simulink model "InverterOnly"  (R2016b)
settings: Solver=ode45  StartTime=0*24*3600  StopTime=3600  MaxStep=60  RelTol=1e-4  EnableMultiTasking=on
libraries: carnot x1, simulink x1
settings Model: Creator=drhf  LastModifiedBy=drhf
settings DataIOCC: LimitDataPoints=on  SaveFormat=Array  SignalLoggingSaveFormat=ModelDataLogs
settings OptimizationCC: ExpressionDepthLimit=2147483647  LifeSpan=inf
settings DebuggingCC: UnderspecifiedInitializationDetection=Classic  MergeDetectMultiDrivingBlocksExec=none  SolverPrmCheckMsg=warning  FcnCallInpInsideContextMsg=warning  StateNameClashWarn=warning  SFUnexpectedBacktrackingDiag=warning  SFNoUnconditionalDefaultTransitionDiag=warning  SFExecutionAtInitializationDiag=none
settings HardwareCC: ProdBitPerPointer=32  ProdBitPerSizeT=32  ProdBitPerPtrDiffT=32  ProdLargestAtomicFloat=None  ProdIntDivRoundTo=Undefined  ProdEndianess=Unspecified  ProdWordSize=32  ProdHWDeviceType=32-bit Generic
settings ModelReferenceCC: PropagateSignalLabelsOutOfModel=off
settings GRTTargetCC: TargetLangStandard=C89/C90 (ANSI)  GeneratePreprocessorConditionals=Disable all  CombineOutputUpdateFcns=off  GRTInterface=on
settings ConfigComp: CovMetricSettings=dw  CovHtmlReporting=on  CovSaveCumulativeToWorkspaceVar=on  CovSaveSingleToWorkspaceVar=on  CovExternalEMLEnable=off

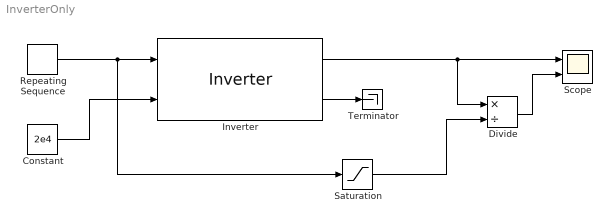
== system InverterOnly ==
  Constant : Constant  Value=2e4
  Divide : Product  Inputs=*/
  Inverter : carnot/Source/Electric_Generator/Inverter  P0=9000  ol=1.2  power_steps=[0 0.05 0.1 0.2 0.3 0.5 1 1.2]  eta_steps=[0 0.924 0.958 0.974 0.979 0.981 0.98 0.95]  standby=1
  Repeating Sequence : simulink/Sources/Repeating Sequence  rep_seq_t=[0 3600]  rep_seq_y=[0 10e3]
  Saturation : Saturate  UpperLimit=inf  LowerLimit=1
  Scope : Scope  NumInputPorts=2
  Terminator : Terminator
  wires:
  Repeating Sequence/1 -> Inverter/1, Saturation/1
  Inverter/1 -> Scope/1, Divide/1
  Divide/1 -> Scope/2
  Inverter/2 -> Terminator/1
  Constant/1 -> Inverter/2
  Saturation/1 -> Divide/2
